simulink model "GreenCraneActualPrints"  (R2025b)
settings: Solver=VariableStepAuto  StartTime=0.0  StopTime=30  RelTol=1e-3
model workspace (MATLAB code in the model file):
  rho = 875
  beta = 1000
  pP = 10e6    (= 10000000)
  pA_Cyl_Initial = 67
  dp0 = 20e5    (= 2000000)
  Q0 = 18/6e4    (= 0.0003)
  Cd = 0.55
  AdMax_SI = Q0/(Cd*(2/rho*dp0)^0.5)    (= 8.06738152241e-06)
  AdMax = AdMax_SI*1e6    (= 8.06738152241)
  Tau_DCV = 0.1
  TauP = 1/(2*pi*5)    (= 0.0318309886184)
  u_dead_up = 0.236
  u_dead_down = 0.206
  spool_dead_up = 1.1182 * u_dead_up   - 0.0325    (= 0.2313952)
  spool_dead_down = 1.1075 * u_dead_down - 0.0416    (= 0.186545)
  p_spool_of_Kv_up = [0.0018653, -0.033672,  0.22033, -0.65618,  0.83411, -0.047269, 0.26252]
  p_spool_of_Kv_down = [0.00098272, -0.017507,  0.11599, -0.34851,  0.41222,  0.17643,  0.2076]
  slope_Kv_up = 0.3410    (= 0.341)
  slope_Kv_down = 0.4248
  Kv_range = linspace(0.09, 4, 10000)
  spool_up = polyval(p_spool_of_Kv_up,   Kv_range)
  spool_down = polyval(p_spool_of_Kv_down, Kv_range)
  u_breakpoints = 0.25:0.05:1.0
  spool_bp_up = 1.1182 * u_breakpoints - 0.0325
  spool_bp_down = 1.1075 * u_breakpoints - 0.0416
  Kv_bp_up = zeros(1, length(u_breakpoints))
  Kv_bp_down = zeros(1, length(u_breakpoints))
  Kv_max_up = Kv_range(idx_max_up)
  Kv_max_down = Kv_range(idx_max_down)
  Kv_unit_conv = sqrt(1e-5) / 6e4
  A_bp_up = (Kv_bp_up   * Kv_unit_conv) / (Cd * sqrt(2/rho))
  A_bp_down = (Kv_bp_down * Kv_unit_conv) / (Cd * sqrt(2/rho))
  A_max_up = (Kv_max_up  * Kv_unit_conv) / (Cd * sqrt(2/rho))
  A_max_down = (Kv_max_down* Kv_unit_conv) / (Cd * sqrt(2/rho))
  orifice_area_down = [1e-9, A_bp_down, A_max_down]
  u_max_pos = 1.05
  control_pos_up = [0, spool_bp_up,   1.1182 * u_max_pos - 0.0325]
  control_pos_down = [0, spool_bp_down, 1.1075 * u_max_pos - 0.0416]
  alpha = 5
  pCr_A = 230e5    (= 23000000)
  dp_open_A = 150e5    (= 15000000)
  Cd_CBV = 0.8
  AdMax_CBV = (60 / 6e4) / sqrt(2/rho * 16e5) / Cd_CBV
  d = 65
  dr = 35
  A = pi*d^2/4    (= 3318.30724035)
  Ar = pi*dr^2/4    (= 962.112750162)
  Aa = A - Ar    (= 2356.19449019)
  h = 500
  L0 = 272
  dx = 0
  L = h + L0 + dx    (= 772)
  m = 75*4 + 20 + 90    (= 410)
  g = 9.81
  MG = m*g    (= 4022.1)
  x_Init = 100
  Cx = 427
  Cz = -1057
  theta_Init = 73.04- 90    (= -16.96)
  thetaDot_Init = 0
  L1 = 3680
  B1 = 100
  H1 = 150
  t1 = 6
  revBasePinDia = 60
  revBasePinLength = 185.5
  rEar = 35
  tEar = 30
  earToCylTop = 52.45
  earToCylBot = 40.62
  cylDia = 75
  cylLength = 682
  rodLength = 565.26
  rodDia = 35
  rodToCyl = 132
  revCylPinDia = 25
  revCylPinLength = 84
  rPiston = 65/2    (= 32.5)
  tPiston = 40
  abx = 564.99
  aby = 133
  L2 = 210
  B2 = 700
  H2 = 300
  dY_PL_Beam = 75
  beam_mass = 415.740    (= 415.74)
  beam_COM = [3216.15, 61.48, 0.00]
  cyl_house_mass = 10.46699
  cyl_house_COM = [260.99, 0.16, 0.00]
  cyl_rod_mass = 4.81658
  cyl_rod_COM = [-292.43, 0.00, 0.00]
  beam_MOI = [17.5673, 453.1288, 442.0275]
  beam_POI = [13.7279, 0.00000, 0.00000]
  cyl_house_MOI = [0.00969, 0.50582, 0.50623]
  cyl_house_POI = [-0.00039, 0.00000, 0.00000]
  cyl_rod_MOI = [0.00142, 0.20919, 0.20942]
  cyl_rod_POI = [0.00000, 0.00000, 0.00000]
  F_C = 609
  v_th = 1e-3    (= 0.001)
  dt = 0.001
  TauF = 0.01
  Kf = 0.0005
  other statements: clear;; for i = 1:length(u_breakpoints); if u_breakpoints(i) <= 0.25; Kv_bp_up(i)   = (spool_bp_up(i)   - spool_dead_up)   / slope_Kv_up;; Kv_bp_down(i) = (spool_bp_down(i) - spool_dead_down) / slope_Kv_down;; else; [~, idx_up]   = min(abs(spool_up   - spool_bp_up(i)));; [~, idx_down] = min(abs(spool_down - spool_bp_down(i)));; Kv_bp_up(i)   = Kv_range(idx_up);; Kv_bp_down(i) = Kv_range(idx_down);; end; end ... (+2)
undefined symbols (not defined in the file): orifice_area_up, X, Y, Z
libraries: sm_lib x41, fl_lib x19, nesl_utility x16, SimscapeFluids_lib x7, slpidlib x1
(part 2 of 2)

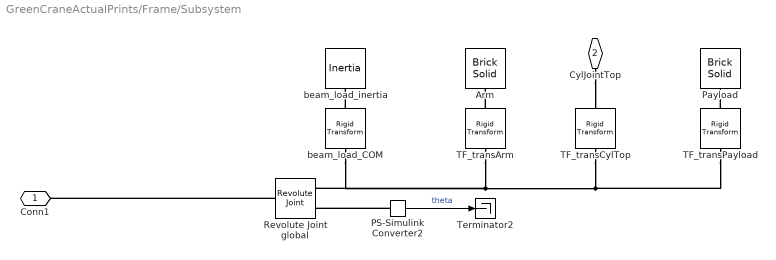
== system GreenCraneActualPrints/Frame/Subsystem ==
  Arm : sm_lib/Body Elements/Brick Solid  BrickDimensions=[L1 H1 B1]  BrickDimensionsUnits=mm  ExportEntireGeometry=off  InertiaType=Custom  BasedOnType=Density  Density=1000  DensityUnits=kg/m^3  Mass=1  MassUnits=kg  CenterOfMass=[0 0 0]  CenterOfMassUnits=m  MomentsOfInertia=[1 1 1]  MomentsOfInertiaUnits=kg*m^2  ProductsOfInertia=[0 0 0]  ProductsOfInertiaUnits=kg*m^2  GraphicType=FromGeometry  MarkerShape=Sphere  MarkerSize=10  GraphicVisPropType=SimpleVisualProperties  GraphicDiffuseColor=[0.3569 0.4157 0.2314]  GraphicOpacity=1  GraphicSpecularColor=[0.5 0.5 0.5 1.0]  GraphicAmbientColor=[0.15 0.15 0.15 1.0]  GraphicEmissiveColor=[0.0 0.0 0.0 1.0]  GraphicShininess=75  DoExposeReferenceFrame=on  SerializedFrames=<Frames/>
  PS-Simulink Converter2 : nesl_utility/PS-Simulink Converter  PhysicalDomain=network_engine_domain  SubClassName=ps_output  LeftPortType=input  RightPortType=output  PseudoPeriodic=off  Frequencies=[]  VectorFormat=inherit  Unit=inherit  AffineConversion=off
  Payload : sm_lib/Body Elements/Brick Solid  BrickDimensions=[L2 H2 B2]  BrickDimensionsUnits=mm  ExportEntireGeometry=off  InertiaType=Custom  BasedOnType=Density  Density=1000  DensityUnits=kg/m^3  Mass=1  MassUnits=kg  CenterOfMass=[0 0 0]  CenterOfMassUnits=m  MomentsOfInertia=[1 1 1]  MomentsOfInertiaUnits=kg*m^2  ProductsOfInertia=[0 0 0]  ProductsOfInertiaUnits=kg*m^2  GraphicType=FromGeometry  MarkerShape=Sphere  MarkerSize=10  GraphicVisPropType=SimpleVisualProperties  GraphicDiffuseColor=[0.8941 0.7922 0.2902]  GraphicOpacity=1  GraphicSpecularColor=[0.5 0.5 0.5 1.0]  GraphicAmbientColor=[0.15 0.15 0.15 1.0]  GraphicEmissiveColor=[0.0 0.0 0.0 1.0]  GraphicShininess=75  DoExposeReferenceFrame=on  SerializedFrames=<Frames/>
  Revolute Joint global : sm_lib/Joints/Revolute Joint  JointMode=Normal  CompositeWrenchDir=FollowerOnBase  CompositeWrenchFrame=BaseFrame  SenseConstraintForce=off  SenseConstraintTorque=off  SenseTotalForce=off  SenseTotalTorque=off  PositionTargetSpecify=on  PositionTargetPriority=High  PositionTargetValue=theta_Init  PositionTargetValueUnits=deg  VelocityTargetSpecify=on  VelocityTargetPriority=High  VelocityTargetValue=thetaDot_Init  VelocityTargetValueUnits=deg/s  EquilibriumPosition=0  EquilibriumPositionUnits=deg  SpringStiffness=0  SpringStiffnessUnits=N*m/deg  DampingCoefficient=0  DampingCoefficientUnits=N*m/(deg/s)  LowerLimitSpecify=off  LowerLimitBound=-90  LowerLimitBoundUnits=deg  LowerLimitStiffness=1e4  LowerLimitStiffnessUnits=N*m/deg  LowerLimitDamping=10  LowerLimitDampingUnits=N*m/(deg/s)  LowerLimitTransitionRegionWidth=0.1  LowerLimitTransitionRegionWidthUnits=deg  UpperLimitSpecify=off  UpperLimitBound=90  UpperLimitBoundUnits=deg  UpperLimitStiffness=1e4  UpperLimitStiffnessUnits=N*m/deg  UpperLimitDamping=10  UpperLimitDampingUnits=N*m/(deg/s)  UpperLimitTransitionRegionWidth=0.1  UpperLimitTransitionRegionWidthUnits=deg  TorqueActuationMode=NoTorque  MotionActuationMode=ComputedMotion  SensePosition=on  SenseVelocity=off  SenseAcceleration=off  SenseTorqueForce=off  SenseLowerLimitTorqueForce=off  SenseUpperLimitTorqueForce=off
  TF_transArm : sm_lib/Frames and Transforms/Rigid Transform  RotationMethod=None  FollAlignAxisA=+X  BaseAlignAxisA=+Y  FollAlignAxisB=+Y  BaseAlignAxisB=+Z  RotationStandardAxis=+Z  RotationAngle=0  RotationAngleUnits=deg  RotationArbitraryAxis=[0 0 1]  RotationSequenceAxes=FollowerAxes  RotationSequence=XYX  RotationSequenceAngles=[0 0 0]  RotationSequenceAnglesUnits=deg  RotationMatrix=[1 0 0;0 1 0;0 0 1]  Quaternion=[1 0 0 0]  TranslationMethod=Cartesian  TranslationCartesianOffset=[L1/2 0 0]  TranslationCartesianOffsetUnits=mm  TranslationStandardAxis=+Z  TranslationStandardOffset=0  TranslationStandardOffsetUnits=m  TranslationROffset=0  TranslationROffsetUnits=m  TranslationThetaOffset=0  TranslationThetaOffsetUnits=deg  TranslationZOffset=0  TranslationZOffsetUnits=m
  TF_transCylTop : sm_lib/Frames and Transforms/Rigid Transform  RotationMethod=None  FollAlignAxisA=+X  BaseAlignAxisA=+Y  FollAlignAxisB=+Y  BaseAlignAxisB=+Z  RotationStandardAxis=+Z  RotationAngle=0  RotationAngleUnits=deg  RotationArbitraryAxis=[0 0 1]  RotationSequenceAxes=FollowerAxes  RotationSequence=XYX  RotationSequenceAngles=[0 0 0]  RotationSequenceAnglesUnits=deg  RotationMatrix=[1 0 0;0 1 0;0 0 1]  Quaternion=[1 0 0 0]  TranslationMethod=Cartesian  TranslationCartesianOffset=[abx -aby 0]  TranslationCartesianOffsetUnits=mm  TranslationStandardAxis=+Z  TranslationStandardOffset=0  TranslationStandardOffsetUnits=m  TranslationROffset=0  TranslationROffsetUnits=m  TranslationThetaOffset=0  TranslationThetaOffsetUnits=deg  TranslationZOffset=0  TranslationZOffsetUnits=m
  TF_transPayload : sm_lib/Frames and Transforms/Rigid Transform  RotationMethod=None  FollAlignAxisA=+X  BaseAlignAxisA=+Y  FollAlignAxisB=+Y  BaseAlignAxisB=+Z  RotationStandardAxis=+Z  RotationAngle=0  RotationAngleUnits=deg  RotationArbitraryAxis=[0 0 1]  RotationSequenceAxes=FollowerAxes  RotationSequence=XYX  RotationSequenceAngles=[0 0 0]  RotationSequenceAnglesUnits=deg  RotationMatrix=[1 0 0;0 1 0;0 0 1]  Quaternion=[1 0 0 0]  TranslationMethod=Cartesian  TranslationCartesianOffset=[L1-L2/2 dY_PL_Beam 0]  TranslationCartesianOffsetUnits=mm  TranslationStandardAxis=+Z  TranslationStandardOffset=0  TranslationStandardOffsetUnits=m  TranslationROffset=0  TranslationROffsetUnits=m  TranslationThetaOffset=0  TranslationThetaOffsetUnits=deg  TranslationZOffset=0  TranslationZOffsetUnits=m
  Terminator2 : Terminator
  beam_load_COM : sm_lib/Frames and Transforms/Rigid Transform  RotationMethod=None  FollAlignAxisA=+X  BaseAlignAxisA=+Y  FollAlignAxisB=+Y  BaseAlignAxisB=+Z  RotationStandardAxis=+Z  RotationAngle=0  RotationAngleUnits=deg  RotationArbitraryAxis=[0 0 1]  RotationSequenceAxes=FollowerAxes  RotationSequence=XYX  RotationSequenceAngles=[0 0 0]  RotationSequenceAnglesUnits=deg  RotationMatrix=[1 0 0;0 1 0;0 0 1]  Quaternion=[1 0 0 0]  TranslationMethod=Cartesian  TranslationCartesianOffset=beam_COM  TranslationCartesianOffsetUnits=mm  TranslationStandardAxis=+Z  TranslationStandardOffset=0  TranslationStandardOffsetUnits=m  TranslationROffset=0  TranslationROffsetUnits=m  TranslationThetaOffset=0  TranslationThetaOffsetUnits=deg  TranslationZOffset=0  TranslationZOffsetUnits=m
  beam_load_inertia : sm_lib/Body Elements/Inertia  InertiaType=Custom  Mass=beam_mass  MassUnits=kg  CenterOfMass=[0 0 0]  CenterOfMassUnits=m  MomentsOfInertia=beam_MOI  MomentsOfInertiaUnits=kg*m^2  ProductsOfInertia=beam_POI  ProductsOfInertiaUnits=kg*m^2  GraphicType=Marker  MarkerShape=Inertia  MarkerSize=20  GraphicVisPropType=SimpleVisualProperties  GraphicDiffuseColor=[0.5 0.5 0.5]  GraphicOpacity=1  GraphicSpecularColor=[0.5 0.5 0.5 1.0]  GraphicAmbientColor=[0.15 0.15 0.15 1.0]  GraphicEmissiveColor=[0.0 0.0 0.0 1.0]  GraphicShininess=75
  Conn1 : PMIOPort  Side=Left
  CylJointTop : PMIOPort  Port=2  Side=Right
  wires:
  PS-Simulink Converter2/1 -> Terminator2/1  "theta"
  connections:
  TF_transArm/LConn1 -- Revolute Joint global/RConn1 -- beam_load_COM/LConn1 -- TF_transPayload/LConn1 -- TF_transCylTop/LConn1
  Revolute Joint global/LConn1 -- Conn1/RConn1
  CylJointTop/RConn1 -- TF_transCylTop/RConn1
  beam_load_COM/RConn1 -- beam_load_inertia/RConn1
  PS-Simulink Converter2/LConn1 -- Revolute Joint global/RConn2
  TF_transArm/RConn1 -- Arm/RConn1
  TF_transPayload/RConn1 -- Payload/RConn1

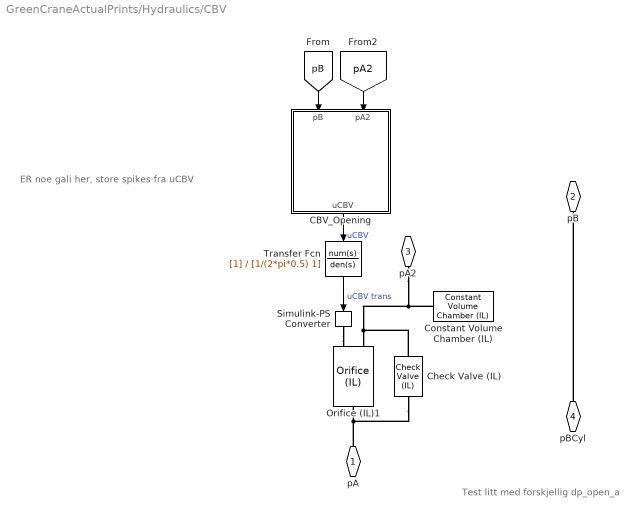
== system GreenCraneActualPrints/Hydraulics/CBV ==
  note: ER noe gali her, store spikes fra uCBV
  note: Test litt med forskjellig dp_open_a
  CBV_Opening : MATLAB Function  TreatAsAtomicUnit=on
  Check Valve (IL) : SimscapeFluids_lib/Isothermal Liquid/Valves & Orifices/Directional Control Valves/Check Valve (IL)  opening_spec=fluids.isothermal_liquid.valves_orifices.enum.PressureOpeningSpec.Linear  pressure_control_spec=fluids.isothermal_liquid.valves_orifices.enum.pressure_control_spec.dp  p_crack_differential=1 bar  p_crack_gauge=0.1 MPa  press_max_differential=2.5 bar  press_max_gauge=0.2 MPa  area_max=AdMax_CBV m^2  area_leak=1e-10 m^2  p_diff_TLU=[0.01 : 0.01 : 0.1] MPa  valve_area_TLU=[1e-10, 1e-05, 2e-05, 3e-05, 4e-05, 5e-05, 6e-05, 7.5e-05, 8.5e-05, .0001] m^2  vol_flow_TLU=[.000358, .045, .11, .191, .284, .39, .505, .63, .764, .905] .* 1e-3 m^3/s  area=inf m^2  Cd=Cd_CBV  Re_c=150  smoothing_factor=0.01  pressure_recovery=false  opening_dynamics=false  tau=0.1 s
      settings: InternalSimscapePortConfiguration="{\"Bottom\":[],\"Left\":[{\"id\":\"A\",\"label\":\"A\",\"type\":\"foundation.isothermal_liquid.isothermal_liquid\"}],\"Right\":[{\"id\":\"B\",\"label\":\"B\",\"type\":\"foundation.isothermal_liquid.isothermal_liquid\"}],\"Top\":[]}"
  Constant Volume Chamber (IL) : fl_lib/Isothermal Liquid/Elements/Constant Volume Chamber (IL)  volume=0.1 l  p_I_specify=on  p_I_priority=High  p_I=pA_Cyl_Initial bar  p_I_nominal_specify=off  p_I_nominal_value=1  p_I_nominal_unit=MPa
      settings: InternalSimscapePortConfiguration="{\"Bottom\":[],\"Left\":[{\"id\":\"A\",\"label\":\"A\",\"type\":\"foundation.isothermal_liquid.isothermal_liquid\"}],\"Right\":[],\"Top\":[]}"
  Orifice (IL)1 : SimscapeFluids_lib/Isothermal Liquid/Valves & Orifices/Orifices/Orifice (IL)  orifice_type=foundation.enum.constant_variable.variable  constant_orifice_spec=fluids.isothermal_liquid.valves_orifices.orifices.enum.constant_orifice_spec.area  variable_orifice_spec=fluids.isothermal_liquid.valves_orifices.orifices.enum.orifice_spec.linear  orifice_area_constant=1e-3 m^2  p_diff_TLU_constant=[-4, -3, -2, -1, -.5, 0, .5, 1, 2, 3, 4] MPa  vol_flow_TLU_constant=[-2.44, -2.12, -1.68, -1.22, -.84, 0, .85, 1.21, 1.7, 2.09, 2.41] .* 1e-3 m^3/s  S_min=0 m  del_S=1 m  open_orientation=fluids.isothermal_liquid.valves_orifices.orifices.enum.orifice_orientation.positive  area_max=AdMax_CBV m^2  area_leak=1e-10 m^2  S_TLU=[0, .002, .004, .007, .017] m  orifice_area_TLU=[1e-09, 2.0352e-07, 4.0736e-05, .00011438, .00034356] m^2  area=inf m^2  Cd=Cd_CBV  Re_c=150  smoothing_factor=0.01  pressure_recovery=false  S_vol_flow_TLU=[0, .002, .004, .007, .017] m  p_diff_TLU=[.3, .5, .7] MPa  vol_flow_TLU=1e-3 * [1.7e-05, 2e-05, 2.6e-05; .0035, .0045, .0053; .7, .9, 1.06; 1.96, 2.5, 3; 6, 7.7, 9.13] m^3/s
      settings: InternalSimscapePortConfiguration="{\"Bottom\":[],\"Left\":[{\"id\":\"A\",\"label\":\"A\",\"type\":\"foundation.isothermal_liquid.isothermal_liquid\"},{\"id\":\"S\",\"label\":\"S\",\"type\":\"input\"}],\"Right\":[{\"id\":\"B\",\"label\":\"B\",\"type\":\"foundation.isothermal_liquid.isothermal_liquid\"}],\"Top\":[]}"
  Simulink-PS Converter : nesl_utility/Simulink-PS Converter  PhysicalDomain=network_engine_domain  SubClassName=ps_input  LeftPortType=input  RightPortType=output  PseudoPeriodic=off  Frequencies=[]  NoiseDistribution=none  NoiseParameters=[]  Unit=1  AffineConversion=off  FilteringAndDerivatives=provide  SimscapeFilterOrder=1  InputFilterTimeConstant=0.001  UdotUserProvided=0
  Transfer Fcn : TransferFcn  Denominator=[1/(2*pi*0.5) 1]
  pA : PMIOPort  Side=Left
  pB : PMIOPort  Port=2  Side=Left
  pA2 : PMIOPort  Port=3  Side=Right
  pBCyl : PMIOPort  Port=4  Side=Right
  wires:
  [pB] -> CBV_Opening/1(pB)
  [pA2] -> CBV_Opening/2(pA2)
  CBV_Opening/1(uCBV) -> Transfer Fcn/1  "uCBV"
  Transfer Fcn/1 -> Simulink-PS Converter/1  "uCBV trans"
  connections:
  Constant Volume Chamber (IL)/LConn1 -- pA2/RConn1 -- Check Valve (IL)/RConn1 -- Orifice (IL)1/LConn1
  Check Valve (IL)/LConn1 -- pA/RConn1 -- Orifice (IL)1/RConn1
  Simulink-PS Converter/RConn1 -- Orifice (IL)1/LConn2
  pBCyl/RConn1 -- pB/RConn1

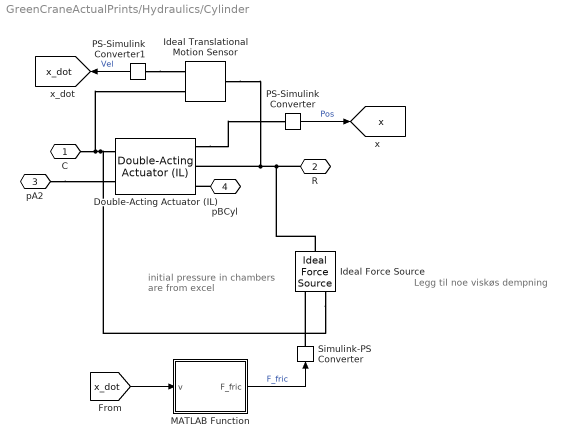
== system GreenCraneActualPrints/Hydraulics/Cylinder ==
  note: Legg til noe viskøs dempning
  note: initial pressure in chambers are from excel
  Double-Acting Actuator (IL) : SimscapeFluids_lib/Isothermal Liquid/Actuators/Double-Acting Actuator (IL)  single_fluid=true  mech_orientation=foundation.enum.MechOrientationTranslational.Positive  piston_area_A=A mm^2  piston_area_B=Aa mm^2  stroke=h mm  dead_volume_A=1e-5 m^3  dead_volume_B=1e-5 m^3  pressure_spec=foundation.enum.pressure_spec.atmospheric  environment_pressure=0.101325 MPa  hardstop_model=simscape.enum.hardstop.smooth  stiff_coeff=1e10 N/m  damping_coeff=150 N*s/m  transition=0.1 mm  coeff_rest=0.7  v_tol=0.001 m/s  f_tol=0.001 N  cushion_A_spec=false  area_plunger_A=1e-4 m^2  length_plunger_A=1e-3 m  area_cushion_orifice_A=1e-6 m^2  area_leak_plunger_A=1e-7 m^2  p_crack_differential_A=0.01 MPa  press_max_differential_A=0.1 MPa  check_valve_area_max_A=1e-4 m^2  check_valve_area_leak_A=1e-10 m^2  smoothing_factor_A=0.01  cushion_B_spec=false  area_plunger_B=1e-4 m^2  length_plunger_B=1e-3 m  area_cushion_orifice_B=1e-6 m^2  area_leak_plunger_B=1e-7 m^2  p_crack_differential_B=0.01 MPa  press_max_differential_B=0.1 MPa  check_valve_area_max_B=1e-4 m^2  check_valve_area_leak_B=1e-10 m^2  smoothing_factor_B=0.01  friction_spec=true  breakaway_Coulomb_ratio=1.2  breakaway_velocity=0.1 m/s  preload_force=20 N  Coulomb_coeff=1e-5 N/Pa  viscous_coeff=100 N*s/m  leakage_spec=false  clearance=1e-4 m  piston_length=0.01 m  displacement_spec=foundation.enum.DisplacementSpec.Calculate  x0=x_Init mm  dynamic_compressibility=true  p0_A=pA_Cyl_Initial bar  p0_B=0.1 bar  p_nominal_A=0.101325 MPa  p_nominal_B=0.101325 MPa
      settings: InternalSimscapePortConfiguration="{\"Bottom\":[],\"Left\":[{\"id\":\"C\",\"label\":\"C\",\"type\":\"foundation.mechanical.translational.translational\"},{\"id\":\"A\",\"label\":\"A\",\"type\":\"foundation.isothermal_liquid.isothermal_liquid\"}],\"Right\":[{\"id\":\"p_out\",\"label\":\"p\",\"type\":\"output\"},{\"id\":\"R\",\"label\":\"R\",\"type\":\"foundation.mechanical.translational.translational\"},{\"id\":\"B\",\"label\":\"B\",\"type\":\"foundation.isothermal_liquid.isothermal_liquid\"}],\"Top\":[]}"
  Ideal Force Source : fl_lib/Mechanical/Mechanical Sources/Ideal Force Source
  Ideal Translational Motion Sensor : fl_lib/Mechanical/Mechanical Sensors/Ideal Translational Motion Sensor  reference=foundation.enum.MeasurementReference.difference  acceleration_port=false  velocity_port=true  position_port=false  offset=0 mm
      settings: InternalSimscapePortConfiguration="{\"Bottom\":[],\"Left\":[{\"id\":\"R\",\"label\":\"R\",\"type\":\"foundation.mechanical.translational.translational\"}],\"Right\":[{\"id\":\"C\",\"label\":\"C\",\"type\":\"foundation.mechanical.translational.translational\"},{\"id\":\"V\",\"label\":\"V\",\"type\":\"output\"}],\"Top\":[]}"
  MATLAB Function : MATLAB Function  TreatAsAtomicUnit=on
  PS-Simulink Converter : nesl_utility/PS-Simulink Converter  PhysicalDomain=network_engine_domain  SubClassName=ps_output  LeftPortType=input  RightPortType=output  PseudoPeriodic=off  Frequencies=[]  VectorFormat=inherit  Unit=inherit  AffineConversion=off
  PS-Simulink Converter1 : nesl_utility/PS-Simulink Converter  PhysicalDomain=network_engine_domain  SubClassName=ps_output  LeftPortType=input  RightPortType=output  PseudoPeriodic=off  Frequencies=[]  VectorFormat=inherit  Unit=inherit  AffineConversion=off
  Simulink-PS Converter : nesl_utility/Simulink-PS Converter  PhysicalDomain=network_engine_domain  SubClassName=ps_input  LeftPortType=input  RightPortType=output  PseudoPeriodic=off  Frequencies=[]  NoiseDistribution=none  NoiseParameters=[]  Unit=1  AffineConversion=off  FilteringAndDerivatives=provide  SimscapeFilterOrder=1  InputFilterTimeConstant=0.001  UdotUserProvided=0
  C : PMIOPort  Side=Right
  R : PMIOPort  Port=2  Side=Right
  pA2 : PMIOPort  Port=3  Side=Right
  pBCyl : PMIOPort  Port=4  Side=Right
  tag scope: x=global, x_dot=global
  wires:
  PS-Simulink Converter1/1 -> [x_dot]  "Vel"
  PS-Simulink Converter/1 -> [x]  "Pos"
  MATLAB Function/1(F_fric) -> Simulink-PS Converter/1  "F_fric"
  [x_dot] -> MATLAB Function/1(v)
  connections:
  C/RConn1 -- Ideal Force Source/RConn2 -- Double-Acting Actuator (IL)/LConn1 -- Ideal Translational Motion Sensor/RConn1
  pBCyl/RConn1 -- Double-Acting Actuator (IL)/RConn3
  PS-Simulink Converter1/LConn1 -- Ideal Translational Motion Sensor/RConn2
  pA2/RConn1 -- Double-Acting Actuator (IL)/LConn2
  Double-Acting Actuator (IL)/RConn1 -- PS-Simulink Converter/LConn1
  Ideal Translational Motion Sensor/LConn1 -- Ideal Force Source/LConn1 -- R/RConn1 -- Double-Acting Actuator (IL)/RConn2
  Simulink-PS Converter/RConn1 -- Ideal Force Source/RConn1

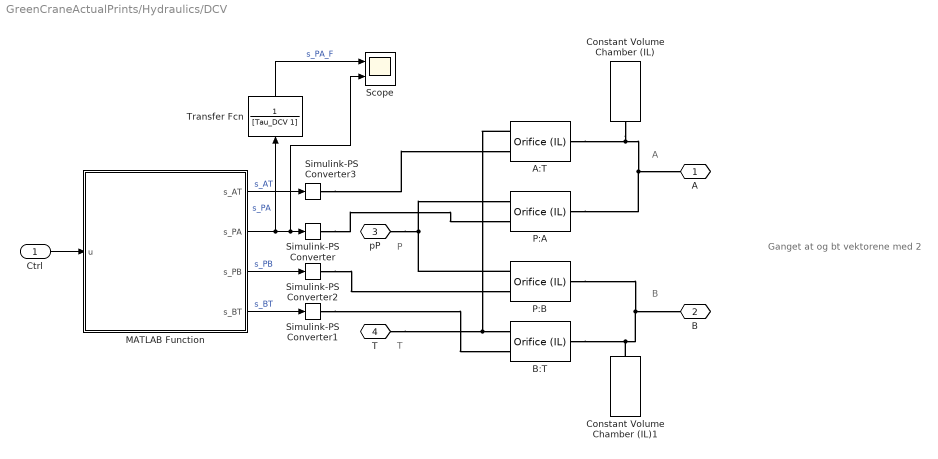
== system GreenCraneActualPrints/Hydraulics/DCV ==
  note: A
  note: B
  note: P
  note: T
  note: Ganget at og bt vektorene med 2
  Ctrl : Inport
  A:T : SimscapeFluids_lib/Isothermal Liquid/Valves & Orifices/Orifices/Orifice (IL)  orifice_type=foundation.enum.constant_variable.variable  constant_orifice_spec=fluids.isothermal_liquid.valves_orifices.orifices.enum.constant_orifice_spec.area  variable_orifice_spec=fluids.isothermal_liquid.valves_orifices.orifices.enum.orifice_spec.table1D_area_opening  orifice_area_constant=1e-3 m^2  p_diff_TLU_constant=[-4, -3, -2, -1, -.5, 0, .5, 1, 2, 3, 4] MPa  vol_flow_TLU_constant=[-2.44, -2.12, -1.68, -1.22, -.84, 0, .85, 1.21, 1.7, 2.09, 2.41] .* 1e-3 m^3/s  S_min=0 m  del_S=5e-3 m  open_orientation=fluids.isothermal_liquid.valves_orifices.orifices.enum.orifice_orientation.positive  area_max=1e-4 m^2  area_leak=1e-10 m^2  S_TLU=control_pos_down m  orifice_area_TLU=orifice_area_down*2 m^2  area=inf m^2  Cd=Cd  Re_c=150  smoothing_factor=0.01  pressure_recovery=false  S_vol_flow_TLU=[0, .002, .004, .007, .017] m  p_diff_TLU=[.3, .5, .7] MPa  vol_flow_TLU=1e-3 * [1.7e-05, 2e-05, 2.6e-05; .0035, .0045, .0053; .7, .9, 1.06; 1.96, 2.5, 3; 6, 7.7, 9.13] m^3/s
      settings: InternalSimscapePortConfiguration="{\"Bottom\":[],\"Left\":[{\"id\":\"A\",\"label\":\"A\",\"type\":\"foundation.isothermal_liquid.isothermal_liquid\"},{\"id\":\"S\",\"label\":\"S\",\"type\":\"input\"}],\"Right\":[{\"id\":\"B\",\"label\":\"B\",\"type\":\"foundation.isothermal_liquid.isothermal_liquid\"}],\"Top\":[]}"
  B:T : SimscapeFluids_lib/Isothermal Liquid/Valves & Orifices/Orifices/Orifice (IL)  orifice_type=foundation.enum.constant_variable.variable  constant_orifice_spec=fluids.isothermal_liquid.valves_orifices.orifices.enum.constant_orifice_spec.area  variable_orifice_spec=fluids.isothermal_liquid.valves_orifices.orifices.enum.orifice_spec.table1D_area_opening  orifice_area_constant=1e-3 m^2  p_diff_TLU_constant=[-4, -3, -2, -1, -.5, 0, .5, 1, 2, 3, 4] MPa  vol_flow_TLU_constant=[-2.44, -2.12, -1.68, -1.22, -.84, 0, .85, 1.21, 1.7, 2.09, 2.41] .* 1e-3 m^3/s  S_min=0 m  del_S=5e-3 m  open_orientation=fluids.isothermal_liquid.valves_orifices.orifices.enum.orifice_orientation.positive  area_max=area_vector_up m^2  area_leak=1e-10 m^2  S_TLU=control_pos_up m  orifice_area_TLU=orifice_area_up*2 m^2  area=inf m^2  Cd=Cd  Re_c=150  smoothing_factor=0.01  pressure_recovery=false  S_vol_flow_TLU=[0, .002, .004, .007, .017] m  p_diff_TLU=[.3, .5, .7] MPa  vol_flow_TLU=1e-3 * [1.7e-05, 2e-05, 2.6e-05; .0035, .0045, .0053; .7, .9, 1.06; 1.96, 2.5, 3; 6, 7.7, 9.13] m^3/s
      settings: InternalSimscapePortConfiguration="{\"Bottom\":[],\"Left\":[{\"id\":\"A\",\"label\":\"A\",\"type\":\"foundation.isothermal_liquid.isothermal_liquid\"},{\"id\":\"S\",\"label\":\"S\",\"type\":\"input\"}],\"Right\":[{\"id\":\"B\",\"label\":\"B\",\"type\":\"foundation.isothermal_liquid.isothermal_liquid\"}],\"Top\":[]}"
  Constant Volume Chamber (IL) : fl_lib/Isothermal Liquid/Elements/Constant Volume Chamber (IL)  volume=0.1 l  p_I_specify=on  p_I_priority=High  p_I=0.1 bar  p_I_nominal_specify=off  p_I_nominal_value=1  p_I_nominal_unit=MPa
      settings: InternalSimscapePortConfiguration="{\"Bottom\":[],\"Left\":[{\"id\":\"A\",\"label\":\"A\",\"type\":\"foundation.isothermal_liquid.isothermal_liquid\"}],\"Right\":[],\"Top\":[]}"
  Constant Volume Chamber (IL)1 : fl_lib/Isothermal Liquid/Elements/Constant Volume Chamber (IL)  volume=0.1 l  p_I_specify=on  p_I_priority=High  p_I=0.1 bar  p_I_nominal_specify=off  p_I_nominal_value=1  p_I_nominal_unit=MPa
      settings: InternalSimscapePortConfiguration="{\"Bottom\":[],\"Left\":[{\"id\":\"A\",\"label\":\"A\",\"type\":\"foundation.isothermal_liquid.isothermal_liquid\"}],\"Right\":[],\"Top\":[]}"
  MATLAB Function : MATLAB Function  TreatAsAtomicUnit=on
  P:A : SimscapeFluids_lib/Isothermal Liquid/Valves & Orifices/Orifices/Orifice (IL)  orifice_type=foundation.enum.constant_variable.variable  constant_orifice_spec=fluids.isothermal_liquid.valves_orifices.orifices.enum.constant_orifice_spec.area  variable_orifice_spec=fluids.isothermal_liquid.valves_orifices.orifices.enum.orifice_spec.table1D_area_opening  orifice_area_constant=1e-3 m^2  p_diff_TLU_constant=[-4, -3, -2, -1, -.5, 0, .5, 1, 2, 3, 4] MPa  vol_flow_TLU_constant=[-2.44, -2.12, -1.68, -1.22, -.84, 0, .85, 1.21, 1.7, 2.09, 2.41] .* 1e-3 m^3/s  S_min=0 m  del_S=1 m  open_orientation=fluids.isothermal_liquid.valves_orifices.orifices.enum.orifice_orientation.positive  area_max=A_max_up m^2  area_leak=1e-10 m^2  S_TLU=control_pos_up m  orifice_area_TLU=orifice_area_up m^2  area=inf m^2  Cd=Cd  Re_c=150  smoothing_factor=0.01  pressure_recovery=false  S_vol_flow_TLU=[0, .002, .004, .007, .017] m  p_diff_TLU=[.3, .5, .7] MPa  vol_flow_TLU=1e-3 * [1.7e-05, 2e-05, 2.6e-05; .0035, .0045, .0053; .7, .9, 1.06; 1.96, 2.5, 3; 6, 7.7, 9.13] m^3/s
      settings: InternalSimscapePortConfiguration="{\"Bottom\":[],\"Left\":[{\"id\":\"A\",\"label\":\"A\",\"type\":\"foundation.isothermal_liquid.isothermal_liquid\"},{\"id\":\"S\",\"label\":\"S\",\"type\":\"input\"}],\"Right\":[{\"id\":\"B\",\"label\":\"B\",\"type\":\"foundation.isothermal_liquid.isothermal_liquid\"}],\"Top\":[]}"
  P:B : SimscapeFluids_lib/Isothermal Liquid/Valves & Orifices/Orifices/Orifice (IL)  orifice_type=foundation.enum.constant_variable.variable  constant_orifice_spec=fluids.isothermal_liquid.valves_orifices.orifices.enum.constant_orifice_spec.area  variable_orifice_spec=fluids.isothermal_liquid.valves_orifices.orifices.enum.orifice_spec.table1D_area_opening  orifice_area_constant=1e-3 m^2  p_diff_TLU_constant=[-4, -3, -2, -1, -.5, 0, .5, 1, 2, 3, 4] MPa  vol_flow_TLU_constant=[-2.44, -2.12, -1.68, -1.22, -.84, 0, .85, 1.21, 1.7, 2.09, 2.41] .* 1e-3 m^3/s  S_min=0 m  del_S=1 m  open_orientation=fluids.isothermal_liquid.valves_orifices.orifices.enum.orifice_orientation.positive  area_max=A_max_down m^2  area_leak=1e-10 m^2  S_TLU=control_pos_down m  orifice_area_TLU=orifice_area_down m^2  area=inf m^2  Cd=Cd  Re_c=150  smoothing_factor=0.01  pressure_recovery=false  S_vol_flow_TLU=[0, .002, .004, .007, .017] m  p_diff_TLU=[.3, .5, .7] MPa  vol_flow_TLU=1e-3 * [1.7e-05, 2e-05, 2.6e-05; .0035, .0045, .0053; .7, .9, 1.06; 1.96, 2.5, 3; 6, 7.7, 9.13] m^3/s
      settings: InternalSimscapePortConfiguration="{\"Bottom\":[],\"Left\":[{\"id\":\"A\",\"label\":\"A\",\"type\":\"foundation.isothermal_liquid.isothermal_liquid\"},{\"id\":\"S\",\"label\":\"S\",\"type\":\"input\"}],\"Right\":[{\"id\":\"B\",\"label\":\"B\",\"type\":\"foundation.isothermal_liquid.isothermal_liquid\"}],\"Top\":[]}"
  Scope : Scope  NumInputPorts=2
      settings: ActiveDisplayYMinimum=-0.13571249999999999  ActiveDisplayYMaximum=1.2214125
  Simulink-PS Converter{,1..3} (4 alike) : nesl_utility/Simulink-PS Converter  PhysicalDomain=network_engine_domain  SubClassName=ps_input  LeftPortType=input  RightPortType=output  PseudoPeriodic=off  Frequencies=[]  NoiseDistribution=none  NoiseParameters=[]  Unit=1  AffineConversion=off  FilteringAndDerivatives=provide  SimscapeFilterOrder=1  InputFilterTimeConstant=0.001  UdotUserProvided=0
  Transfer Fcn : TransferFcn  Denominator=[Tau_DCV 1]
  A : PMIOPort  Side=Left
  B : PMIOPort  Port=2  Side=Left
  pP : PMIOPort  Port=3  Side=Right
  T : PMIOPort  Port=4  Side=Right
  wires:
  MATLAB Function/4(s_BT) -> Simulink-PS Converter1/1  "s_BT"
  MATLAB Function/3(s_PB) -> Simulink-PS Converter2/1  "s_PB"
  MATLAB Function/1(s_AT) -> Simulink-PS Converter3/1  "s_AT"
  Ctrl/1 -> MATLAB Function/1(u)
  Transfer Fcn/1 -> Scope/1  "s_PA_F"
  MATLAB Function/2(s_PA) -> Simulink-PS Converter/1, Scope/2, Transfer Fcn/1  "s_PA"
  connections:
  B:T/RConn1 -- Constant Volume Chamber (IL)1/LConn1 -- P:B/RConn1 -- B/RConn1
  A:T/RConn1 -- Constant Volume Chamber (IL)/LConn1 -- P:A/RConn1 -- A/RConn1
  pP/RConn1 -- P:B/LConn1 -- P:A/LConn1
  T/RConn1 -- A:T/LConn1 -- B:T/LConn1
  Simulink-PS Converter/RConn1 -- P:A/LConn2
  Simulink-PS Converter1/RConn1 -- B:T/LConn2
  Simulink-PS Converter2/RConn1 -- P:B/LConn2
  Simulink-PS Converter3/RConn1 -- A:T/LConn2

== system GreenCraneActualPrints/Hydraulics/Pump ==
  Clock : Clock
  Isothermal Liquid Properties (IL) : fl_lib/Isothermal Liquid/Utilities/Isothermal Liquid Properties (IL)  rho_L_atm=rho kg/m^3  bulk_modulus_model=foundation.enum.bulk_modulus_model.const  beta_gain=6  beta_L_atm=beta MPa  nu_atm=1.0034e-6 m^2/s  p_atm=0.101325 MPa  p_min=1 Pa  properties_range_check=simscape.enum.assert.action.error  air_fraction=0.005  polytropic_index=1.0  rho_g_atm=1.225 kg/m^3  air_dissolution_model=false  p_crit=3 MPa
  Pressure Source (IL) : fl_lib/Isothermal Liquid/Sources/Pressure Source (IL)  source_type=foundation.enum.constant_controlled.controlled  pressure_differential=pP Pa
      settings: InternalSimscapePortConfiguration="{\"Bottom\":[],\"Left\":[{\"id\":\"A\",\"label\":\"A\",\"type\":\"foundation.isothermal_liquid.isothermal_liquid\"},{\"id\":\"P\",\"label\":\"P\",\"type\":\"input\"}],\"Right\":[{\"id\":\"B\",\"label\":\"B\",\"type\":\"foundation.isothermal_liquid.isothermal_liquid\"}],\"Top\":[]}"
  Reservoir (IL) : fl_lib/Isothermal Liquid/Elements/Reservoir (IL)  reservoir_type=foundation.enum.constant_controlled.constant  pressure_spec=foundation.enum.pressure_spec.atmospheric  reservoir_pressure=5 bar
  Simulink-PS Converter : nesl_utility/Simulink-PS Converter  PhysicalDomain=network_engine_domain  SubClassName=ps_input  LeftPortType=input  RightPortType=output  PseudoPeriodic=off  Frequencies=[]  NoiseDistribution=none  NoiseParameters=[]  Unit=1  AffineConversion=off  FilteringAndDerivatives=provide  SimscapeFilterOrder=1  InputFilterTimeConstant=0.001  UdotUserProvided=0
  Solver Configuration : nesl_utility/Solver Configuration  PhysicalDomain=network_engine_domain  SubClassName=solver  LeftPortType=input  RightPortType=generic  Tones=[]  Harmonics=[]  SimulateNoise=off  Profile=off  UseLocalSampling=off  EnableSwitchedLinearOptims=on  FrequencyDomain=off  UseCCode=off  RelTol=0.001  AbsTol=0.001  MinStep=1e-09  ToWorkspace=off  RevertToSquareIcSolve=off  NumHomotopyIterations=100  PhasorMode=off  PhasorModeNumHarmonics=1  ConsistencySolver=NEWTON_XTOL_AFTER_FTOL  IndexReductionMethod=DerivativeReplacement  DoDC=off  ResidualTolerance=1e-09  ConsistencyTolSource=GLOBAL  ConsistencyAbsTol=0.001  ConsistencyRelTol=0.001  ConsistencyTolFactor=0.001  UseLocalSolver=off  LocalSolverChoice=NE_BACKWARD_EULER_ADVANCER  ResolveIndetEquations=on  FunctionEvalNumThread=1  LocalSolverSampleTime=0.001  DoFixedCost=off  MaxNonlinIter=3  MaxModeIter=2  ComputeImpulses=off  ImpulseIterations=2  LinearAlgebra=auto  LinearAlgebraNumThread=0  EquationFormulation=NE_TIME_EF  DelaysMemoryBudget=1024  AutomaticFiltering=on  FilteringTimeConstant=0.001  PartitionStorageMethod=AS_NEEDED  PartitionMemoryBudget=1024  PartitionMethod=ROBUST  MultibodyUseLocalSolver=off  MultibodyLocalSolverChoice=ODE1  MultibodyLocalSolverSampleTime=0.001
  Variable Pressure : MATLAB Function  TreatAsAtomicUnit=on
  pP : PMIOPort  Side=Left
  wires:
  Variable Pressure/1(y) -> Simulink-PS Converter/1
  Clock/1 -> Variable Pressure/1(u)
  connections:
  Solver Configuration/RConn1 -- Isothermal Liquid Properties (IL)/RConn1 -- Reservoir (IL)/LConn1 -- Pressure Source (IL)/LConn1
  Pressure Source (IL)/RConn1 -- pP/RConn1
  Simulink-PS Converter/RConn1 -- Pressure Source (IL)/LConn2

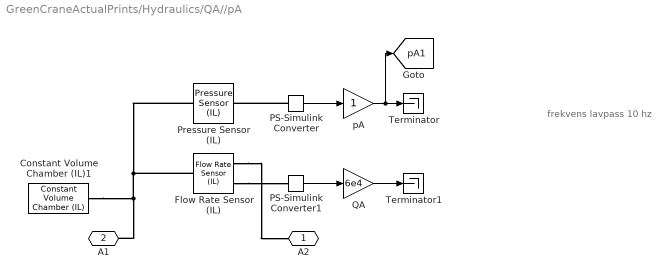
== system GreenCraneActualPrints/Hydraulics/QA//pA ==
  note: frekvens lavpass 10 hz
  Constant Volume Chamber (IL)1 : fl_lib/Isothermal Liquid/Elements/Constant Volume Chamber (IL)  volume=1 l  p_I_specify=on  p_I_priority=High  p_I=0.1 bar  p_I_nominal_specify=off  p_I_nominal_value=1  p_I_nominal_unit=MPa
      settings: InternalSimscapePortConfiguration="{\"Bottom\":[],\"Left\":[{\"id\":\"A\",\"label\":\"A\",\"type\":\"foundation.isothermal_liquid.isothermal_liquid\"}],\"Right\":[],\"Top\":[]}"
  Flow Rate Sensor (IL) : fl_lib/Isothermal Liquid/Sensors/Flow Rate Sensor (IL)  sensor_type=foundation.enum.mass_volumetric_sensor.volumetric
      settings: InternalSimscapePortConfiguration="{\"Bottom\":[],\"Left\":[{\"id\":\"A\",\"label\":\"A\",\"type\":\"foundation.isothermal_liquid.isothermal_liquid\"}],\"Right\":[{\"id\":\"B\",\"label\":\"B\",\"type\":\"foundation.isothermal_liquid.isothermal_liquid\"},{\"id\":\"V\",\"label\":\"V\",\"type\":\"output\"}],\"Top\":[]}"
  PS-Simulink Converter : nesl_utility/PS-Simulink Converter  PhysicalDomain=network_engine_domain  SubClassName=ps_output  LeftPortType=input  RightPortType=output  PseudoPeriodic=off  Frequencies=[]  VectorFormat=inherit  Unit=inherit  AffineConversion=off
  PS-Simulink Converter1 : nesl_utility/PS-Simulink Converter  PhysicalDomain=network_engine_domain  SubClassName=ps_output  LeftPortType=input  RightPortType=output  PseudoPeriodic=off  Frequencies=[]  VectorFormat=inherit  Unit=inherit  AffineConversion=off
  Pressure Sensor (IL) : fl_lib/Isothermal Liquid/Sensors/Pressure Sensor (IL)  pressure_measure=foundation.enum.pressure_measure.gauge
      settings: InternalSimscapePortConfiguration="{\"Bottom\":[],\"Left\":[{\"id\":\"A\",\"label\":\"A\",\"type\":\"foundation.isothermal_liquid.isothermal_liquid\"}],\"Right\":[{\"id\":\"Pg\",\"label\":\"Pg\",\"type\":\"output\"}],\"Top\":[]}"
  QA : Gain  Gain=6e4
  Terminator : Terminator
  Terminator1 : Terminator
  pA : Gain
  A2 : PMIOPort  Side=Left
  A1 : PMIOPort  Port=2  Side=Right
  tag scope: pA1=global
  wires:
  QA/1 -> Terminator1/1
  pA/1 -> [pA1], Terminator/1
  PS-Simulink Converter/1 -> pA/1
  PS-Simulink Converter1/1 -> QA/1
  connections:
  Flow Rate Sensor (IL)/RConn2 -- PS-Simulink Converter1/LConn1
  Constant Volume Chamber (IL)1/LConn1 -- Pressure Sensor (IL)/LConn1 -- Flow Rate Sensor (IL)/LConn1 -- A1/RConn1
  PS-Simulink Converter/LConn1 -- Pressure Sensor (IL)/RConn1
  Flow Rate Sensor (IL)/RConn1 -- A2/RConn1

== system GreenCraneActualPrints/Hydraulics/pA Cylinder sensor ==
  Constant Volume Chamber (IL) : fl_lib/Isothermal Liquid/Elements/Constant Volume Chamber (IL)  volume=0.001 m^3  p_I_specify=on  p_I_priority=High  p_I=pA_Cyl_Initial bar  p_I_nominal_specify=off  p_I_nominal_value=1  p_I_nominal_unit=MPa
      settings: InternalSimscapePortConfiguration="{\"Bottom\":[],\"Left\":[{\"id\":\"A\",\"label\":\"A\",\"type\":\"foundation.isothermal_liquid.isothermal_liquid\"}],\"Right\":[],\"Top\":[]}"
  PS-Simulink Converter : nesl_utility/PS-Simulink Converter  PhysicalDomain=network_engine_domain  SubClassName=ps_output  LeftPortType=input  RightPortType=output  PseudoPeriodic=off  Frequencies=[]  VectorFormat=inherit  Unit=inherit  AffineConversion=off
  Pressure Sensor (IL) : fl_lib/Isothermal Liquid/Sensors/Pressure Sensor (IL)  pressure_measure=foundation.enum.pressure_measure.gauge
      settings: InternalSimscapePortConfiguration="{\"Bottom\":[],\"Left\":[{\"id\":\"A\",\"label\":\"A\",\"type\":\"foundation.isothermal_liquid.isothermal_liquid\"}],\"Right\":[{\"id\":\"Pg\",\"label\":\"Pg\",\"type\":\"output\"}],\"Top\":[]}"
  Terminator : Terminator
  pA2 : Gain
  1 : PMIOPort  Side=Left
  tag scope: pA2=global
  wires:
  PS-Simulink Converter/1 -> pA2/1
  pA2/1 -> [pA2], Terminator/1
  connections:
  PS-Simulink Converter/LConn1 -- Pressure Sensor (IL)/RConn1
  Pressure Sensor (IL)/LConn1 -- Constant Volume Chamber (IL)/LConn1 -- 1/RConn1

== system GreenCraneActualPrints/Hydraulics/pB ==
  Constant Volume Chamber (IL)1 : fl_lib/Isothermal Liquid/Elements/Constant Volume Chamber (IL)  volume=1 l  p_I_specify=on  p_I_priority=High  p_I=0.1 bar  p_I_nominal_specify=off  p_I_nominal_value=1  p_I_nominal_unit=MPa
      settings: InternalSimscapePortConfiguration="{\"Bottom\":[],\"Left\":[{\"id\":\"A\",\"label\":\"A\",\"type\":\"foundation.isothermal_liquid.isothermal_liquid\"}],\"Right\":[],\"Top\":[]}"
  PS-Simulink Converter2 : nesl_utility/PS-Simulink Converter  PhysicalDomain=network_engine_domain  SubClassName=ps_output  LeftPortType=input  RightPortType=output  PseudoPeriodic=off  Frequencies=[]  VectorFormat=inherit  Unit=inherit  AffineConversion=off
  Pressure Sensor (IL)1 : fl_lib/Isothermal Liquid/Sensors/Pressure Sensor (IL)  pressure_measure=foundation.enum.pressure_measure.gauge
      settings: InternalSimscapePortConfiguration="{\"Bottom\":[],\"Left\":[{\"id\":\"A\",\"label\":\"A\",\"type\":\"foundation.isothermal_liquid.isothermal_liquid\"}],\"Right\":[{\"id\":\"Pg\",\"label\":\"Pg\",\"type\":\"output\"}],\"Top\":[]}"
  Terminator : Terminator
  pB : Gain
  1 : PMIOPort  Side=Left
  tag scope: pB=global
  wires:
  PS-Simulink Converter2/1 -> pB/1
  pB/1 -> [pB], Terminator/1
  connections:
  PS-Simulink Converter2/LConn1 -- Pressure Sensor (IL)1/RConn1
  1/RConn1 -- Pressure Sensor (IL)1/LConn1 -- Constant Volume Chamber (IL)1/LConn1

== system GreenCraneActualPrints/Hydraulics/pP ==
  PS-Simulink Converter3 : nesl_utility/PS-Simulink Converter  PhysicalDomain=network_engine_domain  SubClassName=ps_output  LeftPortType=input  RightPortType=output  PseudoPeriodic=off  Frequencies=[]  VectorFormat=inherit  Unit=inherit  AffineConversion=off
  Pressure Sensor (IL)2 : fl_lib/Isothermal Liquid/Sensors/Pressure Sensor (IL)  pressure_measure=foundation.enum.pressure_measure.gauge
      settings: InternalSimscapePortConfiguration="{\"Bottom\":[],\"Left\":[{\"id\":\"A\",\"label\":\"A\",\"type\":\"foundation.isothermal_liquid.isothermal_liquid\"}],\"Right\":[{\"id\":\"Pg\",\"label\":\"Pg\",\"type\":\"output\"}],\"Top\":[]}"
  Terminator : Terminator
  pP : Gain
  1 : PMIOPort  Side=Left
  tag scope: pP=global
  wires:
  PS-Simulink Converter3/1 -> pP/1
  pP/1 -> [pP], Terminator/1
  connections:
  PS-Simulink Converter3/LConn1 -- Pressure Sensor (IL)2/RConn1
  Pressure Sensor (IL)2/LConn1 -- 1/RConn1

== matlab function GreenCraneActualPrints/Hydraulics/CBV/CBV_Opening ==
  data: pB input; pA2 input; uCBV output; pCr_A parameter; dp_open_A parameter; alpha parameter
function uCBV = fcn(pB,pA2,pCr_A, dp_open_A, alpha)

uCBV = (alpha*pB + pA2 - pCr_A) / dp_open_A;
if uCBV < 0
    uCBV = 0;
elseif uCBV > 1
    uCBV = 1;
end

%Jobbe med denne formuleringen, finn kilder

% kjør tester for å finne delta p open og crack pressure. bruk delta p der
% vi har linjær sammenheng.

% crack kjør nedover med ramp til transduser sier ifra om bevegelse, må
% finne ut hva som gir crack pressure og hvor mange trykk som påvirker
% crack ventilen.

%Den er mulig ventilert luft eller tank, så vi skal mulig ikke ha med
%(alpha +1)*pA siden vi har ventilert

== matlab function GreenCraneActualPrints/Control system/Feed forward/sinus_func ==
  data: t input; x_ref output; x_dot_ref output
function [x_ref, x_dot_ref] = fcn(t)
    a_max = 0.150;
    x0    = 0.250;
    f0    = 0.05;     % start frequency (Hz)
    k     = 0.01;     % rate of frequency increase (Hz/s) — tune this

    f   = f0 + k*t;                         % instantaneous frequency
    phi = 2*pi*(f0*t + 0.5*k*t*t);          % integrated phase

    x_ref     = x0 - a_max * cos(phi);
    x_dot_ref = a_max * 2*pi*f * sin(phi);
end


% function [x_ref, x_dot_ref] = fcn(t)
% a_max = 0.150;  % amplitude (half of 300mm travel)
% f     = 0.05;   % frequency
% x0    = 0.250;  % center of 100mm to 400mm range twincat 0.2 ikke 0.25, jeg trenger 0.25 for at start er 0.1m
% x_ref     = x0 - a_max * cos(2*pi*f*t);
% x_dot_ref = a_max * 2*pi*f * sin(2*pi*f*t);

== matlab function GreenCraneActualPrints/Control system/Feed forward/ff_func ==
  data: pA1 input; u_FF output; dP output; Q_req output; pB input; pP input; x_dot_ref input; A parameter; Aa parameter; spool_dead_up parameter; spool_dead_down parameter; slope_Kv_up parameter; slope_Kv_down parameter
function [u_FF, dP, Q_req] = valveFeedForward(pA1, pB, pP, x_dot_ref, A, Aa, spool_dead_up, spool_dead_down, slope_Kv_up, slope_Kv_down)

% Areas from mm^2 to m^2
A  = A  * 1e-6;
Aa = Aa * 1e-6;

dP_min = 1e5;
Kv_conv = sqrt(1e-5) / 6e4; % L/min/sqrt(bar) -> m^3/s/sqrt(Pa)

if x_dot_ref > 0
    % Extension
    Q_req = A * x_dot_ref;
    dP    = max(pP - pA1, dP_min);
    dir   = 1;

    Kv_ref = (Q_req / sqrt(dP)) / Kv_conv;

    if Kv_ref < 0.1
        u_spool = spool_dead_up + slope_Kv_up * Kv_ref;
    else
        u_spool = 0.0018653*Kv_ref^6 - 0.033672*Kv_ref^5 + 0.22033*Kv_ref^4 - 0.65618*Kv_ref^3  + 0.83411*Kv_ref^2  - 0.047269*Kv_ref + 0.26252;
    end
    u_mag = (u_spool + 0.0325) / 1.1182;

elseif x_dot_ref < 0
    % Retraction
    Q_req = Aa * abs(x_dot_ref);
    dP    = max(pP - pB, dP_min);
    dir   = -1;

    Kv_ref = (Q_req / sqrt(dP)) / Kv_conv;

    if Kv_ref < 0.1
        u_spool = spool_dead_down + slope_Kv_down * Kv_ref;
    else
        u_spool = 0.00098272*Kv_ref^6 - 0.017507*Kv_ref^5 + 0.11599*Kv_ref^4 - 0.34851*Kv_ref^3   + 0.41222*Kv_ref^2  + 0.17643*Kv_ref + 0.2076;
    end
    u_mag = (u_spool + 0.0416) / 1.1075;

else
    u_FF  = 0;
    dP    = 0;
    Q_req = 0;
    return
end

u_FF = dir * max(min(u_mag, 1), -1);
end

== matlab function GreenCraneActualPrints/Hydraulics/DCV/MATLAB Function ==
  data: s_AT output; s_PA output; s_PB output; s_BT output; u input; u_dead_up parameter; u_dead_down parameter
function [s_AT, s_PA, s_PB, s_BT] = dcv_spool(u, u_dead_up, u_dead_down)

if u > u_dead_up
    % Extending: PA and BT open
    s_PA = 1.1182 * u - 0.0325;
    s_BT = 1.1182 * u - 0.0325;
    s_PB = 0;
    s_AT = 0;
elseif u < -u_dead_down
    % Retracting: PB and AT open
    s_PA = 0;
    s_BT = 0;
    s_PB = 1.1075 * abs(u) - 0.0416;
    s_AT = 1.1075 * abs(u) - 0.0416;
else
    % Deadband: all at leakage
    s_PA = 0;
    s_BT = 0;
    s_PB = 0;
    s_AT = 0;
end

== matlab function GreenCraneActualPrints/Hydraulics/Cylinder/MATLAB Function ==
  data: v input; F_fric output; v_th parameter; F_C parameter
function F_fric = fcn(v, v_th, F_C)
    F_fric = - F_C * tanh(v / v_th);
end

== matlab function GreenCraneActualPrints/Hydraulics/Pump/Variable Pressure ==
  data: u input; y output
function y = fcn(u)
    % Mean pressure — steps
    if u < 35
        p_mean = 850e5;
    elseif u < 36
        p_mean = 850e5;
    else
        p_mean = 850e5;
    end

    % Smooth pseudo-random variation around the mean
    amp = 5e5;  % ±5 bar variation — tune as needed
    variation = amp * ( sin(0.37*u + 1.2) + sin(0.91*u + 0.4) + sin(1.73*u + 2.1) ) / 3;

    y = p_mean; %+ variation;
end

== matlab function GreenCraneActualPrints/Control system/Pressure Gradient Feedback/MATLAB Function ==
  data: u_FF input; pA_Cyl input; pB input; px output; x_dot_ref input; enable output
function [px, enable] = selectPressure(u_FF, pA_Cyl, pB, x_dot_ref)

% Always pass real pressure to downstream derivative — never artificial zero
if u_FF >= 0
    px = pA_Cyl;   % extension uses bore-side
else
    px = -pB;       % retraction uses rod-side (change to pA_Cyl if preferred) pB needs negative sign. But works worse
end

% Enable feedback only when motion is sufficiently active
if (u_FF > 0 && x_dot_ref > 0.005) || (u_FF < 0 && x_dot_ref < -0.005)
    enable = 1;
else
    enable = 0;
end
end

% function px = selectPressure(u_FF, pA_Cyl, pB, x_dot_ref)
% if u_FF > 0 && x_dot_ref > 0.01
%     px = pA_Cyl;   % extension
% elseif u_FF < 0 && x_dot_ref < -0.01
%     px = pA_Cyl;   % retraction also uses pA_Cyl mulig test -pb
% else
%     px = 0;
% end
